simulink model "KarnoppEventDet"  (R2018b)
settings: Solver=VariableStepAuto  StartTime=0.0  StopTime=10.0  RelTol=1e-3
libraries: simulink x1
settings Model: Creator=Kjetk  LastModifiedBy=Kjetk

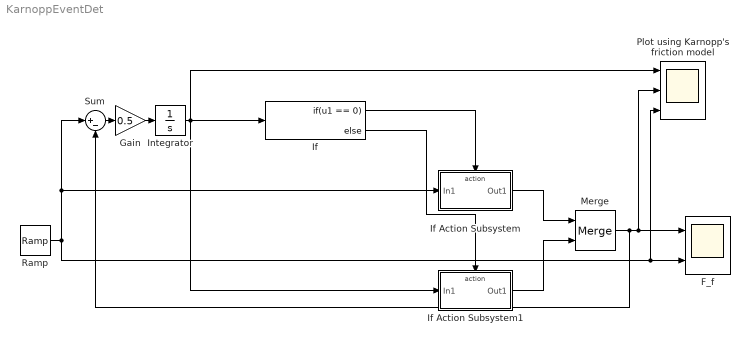
== system KarnoppEventDet ==
  "F_f " : Scope  NumInputPorts=2
  Gain : Gain  Gain=0.5
  If : If  IfExpression=u1 == 0
  If Action Subsystem : Subsystem  TreatAsAtomicUnit=on
  If Action Subsystem1 : Subsystem  TreatAsAtomicUnit=on
  Integrator : Integrator
  Merge : Merge
  "Plot using Karnopp's friction model " : Scope  NumInputPorts=3
  Ramp : simulink/Sources/Ramp  slope=1  start=0  InitialOutput=0
  Sum : Sum  Inputs=|+-
  wires:
  If/2 -> If Action Subsystem1/Action
  If/1 -> If Action Subsystem/Action
  Ramp/1 -> If Action Subsystem/1(In1), Sum/1, "Plot using Karnopp's friction model "/3, "F_f "/2
  Integrator/1 -> If/1, "Plot using Karnopp's friction model "/1, If Action Subsystem1/1(In1)
  If Action Subsystem/1(Out1) -> Merge/1
  If Action Subsystem1/1(Out1) -> Merge/2
  Merge/1 -> "Plot using Karnopp's friction model "/2, "F_f "/1, Sum/2
  Sum/1 -> Gain/1
  Gain/1 -> Integrator/1

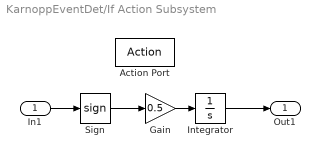
== system KarnoppEventDet/If Action Subsystem ==
  In1 : Inport
  Action Port : ActionPort  ActionType=then
  Gain : Gain  Gain=0.5
  Integrator : Integrator
  Sign : Signum
  Out1 : Outport
  wires:
  In1/1 -> Sign/1
  Sign/1 -> Gain/1
  Gain/1 -> Integrator/1
  Integrator/1 -> Out1/1

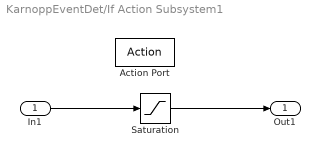
== system KarnoppEventDet/If Action Subsystem1 ==
  In1 : Inport
  Action Port : ActionPort  ActionType=else
  Saturation : Saturate  UpperLimit=4  LowerLimit=-4
  Out1 : Outport
  wires:
  In1/1 -> Saturation/1
  Saturation/1 -> Out1/1
